simulink model "fuzzy"  (R2015a)
settings: Solver=ode45  StartTime=0.0  StopTime=inf  RelTol=1e-3
model workspace (MAT data in the model file):
  SL_ROS_VariableLengthArrays_MaxSizes.CommonInfo.ArrayTruncateAction = 'EmitWarning'
  SL_ROS_VariableLengthArrays_MaxSizes.MsgTypeMap = containers.Map
  SL_ROS_VariableLengthArrays_MaxSizes.MsgTypeMap.serialization.keys = {'sensor_msgs/LaserScan'}
  SL_ROS_VariableLengthArrays_MaxSizes.MsgTypeMap.serialization.values{1}(1).PropertyName = 'Ranges'
  SL_ROS_VariableLengthArrays_MaxSizes.MsgTypeMap.serialization.values{1}(1).DataType = 'single'
  SL_ROS_VariableLengthArrays_MaxSizes.MsgTypeMap.serialization.values{1}(1).MaxLength = 180
  SL_ROS_VariableLengthArrays_MaxSizes.MsgTypeMap.serialization.values{1}(2).PropertyName = 'Intensities'
  SL_ROS_VariableLengthArrays_MaxSizes.MsgTypeMap.serialization.values{1}(2).DataType = 'single'
  SL_ROS_VariableLengthArrays_MaxSizes.MsgTypeMap.serialization.values{1}(2).MaxLength = 128
  SL_ROS_VariableLengthArrays_MaxSizes.MsgTypeMap.serialization.uniformity = 0
  SL_ROS_VariableLengthArrays_MaxSizes.MsgTypeMap.serialization.keyType = 'char'
  SL_ROS_VariableLengthArrays_MaxSizes.MsgTypeMap.serialization.valueType = 'any'
libraries: dspstat3 x6, robotlib x2, fuzblock x1, aerolibutil x1, aerolibtransform2 x1, simulink_extras x1
settings Model: Creator=root  LastModifiedBy=tcoelho

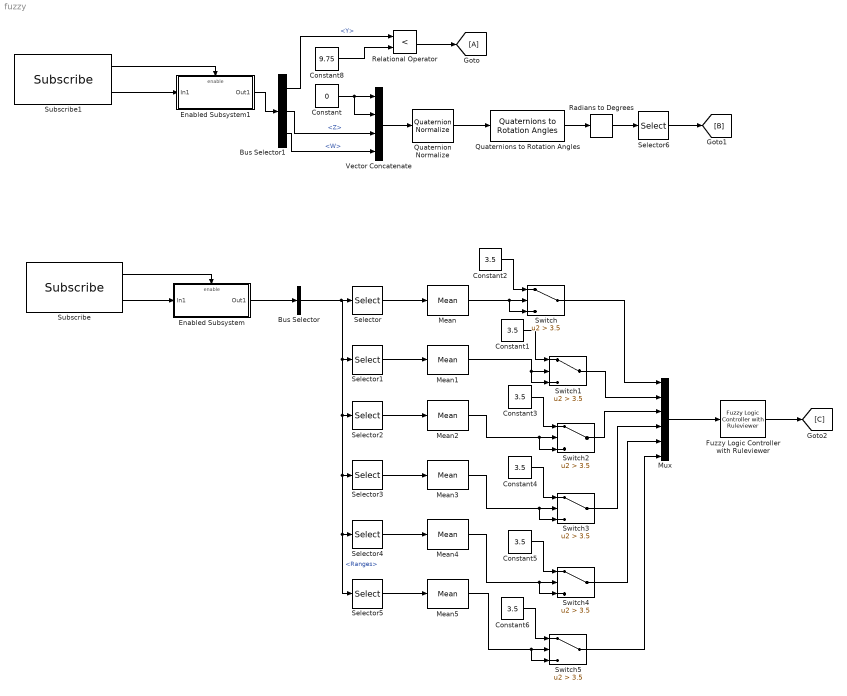
== system fuzzy ==
  Bus Selector : BusSelector  OutputSignals=Ranges
  Bus Selector1 : BusSelector  OutputSignals=Pose.Position.Y,Pose.Orientation.Z,Pose.Orientation.W
  Constant : Constant  Value=0
  Constant{1..6} (6 alike) : Constant  Value=3.5
  Constant8 : Constant  Value=9.75
  Enabled Subsystem : Subsystem  TreatAsAtomicUnit=on
  Enabled Subsystem1 : Subsystem  TreatAsAtomicUnit=on
  Fuzzy Logic Controller with Ruleviewer : fuzblock/Fuzzy Logic  Controller  with Ruleviewer  fismatrix=desvio  Ts=0.5
  Mean{,1..5} (6 alike) : dspstat3/Mean  run=off  reset_popup=None  InputProcessing=Columns as channels (frame based)  directionMode=Entire input  dimension=1  treatSBRowAsCol=off  roiEnable=off  roiType=Rectangles  roiPortion=Entire ROI  roiOutput=Individual statistics for each ROI  roiFlag=off  outputDataTypeStr=Inherit: Same as accumulator  outputLastDataTypeStr=Inherit: Same as accumulator  outputMin=[]  outputMax=[]  roundingMode=Floor  overflowMode=off
  Mux : Mux  Inputs=6
  Quaternion Normalize : aerolibutil/Quaternion Normalize
  Quaternions to Rotation Angles : aerolibtransform2/Quaternions to Rotation Angles  rotationOrder=ZYX
  Radians to Degrees : simulink_extras/Transformations/Radians to Degrees
  Relational Operator : RelationalOperator  Operator=<  OutDataTypeStr=boolean
  Selector : Selector  InputPortWidth=180  Indices=[1:30]
  Selector1 : Selector  InputPortWidth=180  Indices=[31:60]
  Selector2 : Selector  InputPortWidth=180  Indices=[61:90]
  Selector3 : Selector  InputPortWidth=180  Indices=[91:120]
  Selector4 : Selector  InputPortWidth=180  Indices=[121:150]
  Selector5 : Selector  InputPortWidth=180  Indices=[151:180]
  Selector6 : Selector  InputPortWidth=3  Indices=[3]
  Subscribe : robotlib/Subscribe  SourceLibraryInfo=This block requires Robotics System Toolbox  topicSource=Select from ROS network  topic=/RosAria/laser  messageType=sensor_msgs/LaserScan  sampleTime=-1  messageQueueLength=1
  Subscribe1 : robotlib/Subscribe  SourceLibraryInfo=This block requires Robotics System Toolbox  topicSource=Select from ROS network  topic=/RosAria/pose  messageType=geometry_msgs/PoseStamped  sampleTime=-1  messageQueueLength=1
  Switch{,1..5} (6 alike) : Switch  Criteria=u2 > Threshold  Threshold=3.5
  Vector Concatenate : Concatenate  NumInputs=4
  wires:
  Subscribe/2 -> Enabled Subsystem/1(In1)
  Subscribe/1 -> Enabled Subsystem/Enable
  Enabled Subsystem/1(Out1) -> Bus Selector/1
  Bus Selector/1 -> Selector5/1, Selector4/1, Selector3/1, Selector2/1, Selector1/1, Selector/1  "<Ranges>"
  Selector/1 -> Mean/1
  Selector1/1 -> Mean1/1
  Selector2/1 -> Mean2/1
  Selector3/1 -> Mean3/1
  Selector4/1 -> Mean4/1
  Selector5/1 -> Mean5/1
  Mean/1 -> Switch/3, Switch/2
  Constant2/1 -> Switch/1
  Mean1/1 -> Switch1/3, Switch1/2
  Constant1/1 -> Switch1/1
  Mean2/1 -> Switch2/3, Switch2/2
  Constant3/1 -> Switch2/1
  Mean3/1 -> Switch3/3, Switch3/2
  Constant4/1 -> Switch3/1
  Mean4/1 -> Switch4/3, Switch4/2
  Constant5/1 -> Switch4/1
  Mean5/1 -> Switch5/3, Switch5/2
  Constant6/1 -> Switch5/1
  Mux/1 -> Fuzzy Logic Controller with Ruleviewer/1
  Switch/1 -> Mux/1
  Switch1/1 -> Mux/2
  Switch2/1 -> Mux/3
  Switch3/1 -> Mux/4
  Switch4/1 -> Mux/5
  Switch5/1 -> Mux/6
  Subscribe1/1 -> Enabled Subsystem1/Enable
  Subscribe1/2 -> Enabled Subsystem1/1(In1)
  Enabled Subsystem1/1(Out1) -> Bus Selector1/1
  Fuzzy Logic Controller with Ruleviewer/1 -> [C]
  Bus Selector1/1 -> Relational Operator/1  "<Y>"
  Bus Selector1/2 -> Vector Concatenate/3  "<Z>"
  Bus Selector1/3 -> Vector Concatenate/4  "<W>"
  Vector Concatenate/1 -> Quaternion Normalize/1
  Quaternion Normalize/1 -> Quaternions to Rotation Angles/1
  Quaternions to Rotation Angles/1 -> Radians to Degrees/1
  Constant/1 -> Vector Concatenate/2, Vector Concatenate/1
  Constant8/1 -> Relational Operator/2
  Relational Operator/1 -> [A]
  Selector6/1 -> [B]
  Radians to Degrees/1 -> Selector6/1

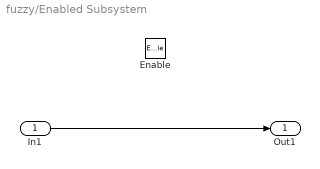
== system fuzzy/Enabled Subsystem ==
  In1 : Inport
  Enable : EnablePort
  Out1 : Outport
  wires:
  In1/1 -> Out1/1

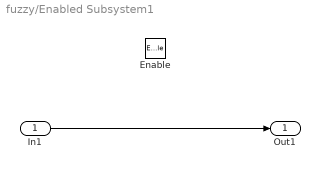
== system fuzzy/Enabled Subsystem1 ==
  In1 : Inport
  Enable : EnablePort
  Out1 : Outport
  wires:
  In1/1 -> Out1/1
